simulink subsystem "digitalOutputs"  (R2023b)
settings: Solver=VariableStepAuto  StartTime=0.0  StopTime=10.0  RelTol=1e-3
settings Model: Creator=serga  LastModifiedBy=serga

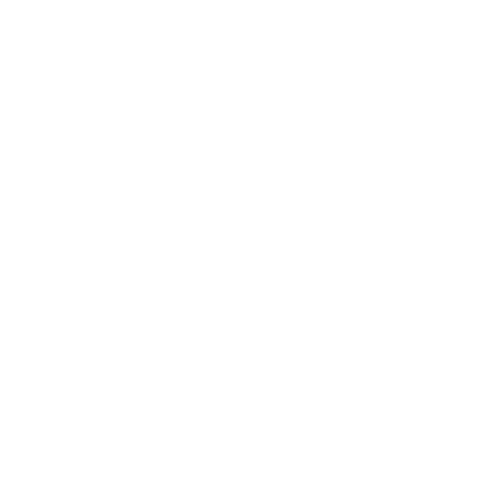
[thumbnail: Simulink's stored preview of the top-level diagram]
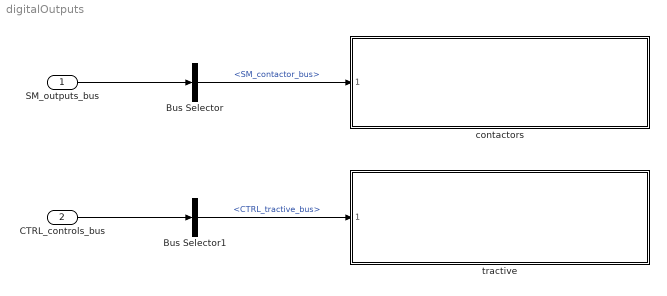
== system digitalOutputs ==
  SM_outputs_bus : Inport
  CTRL_controls_bus : Inport  Port=2
  Bus Selector : BusSelector  OutputSignals=SM_contactor_bus
  Bus Selector1 : BusSelector  OutputSignals=CTRL_tractive_bus
  contactors : Subsystem  ReferencedSubsystem=contactors
  tractive : Subsystem  ReferencedSubsystem=tractive
  wires:
  Bus Selector/1 -> contactors/1  "<SM_contactor_bus>"
  SM_outputs_bus/1 -> Bus Selector/1
  CTRL_controls_bus/1 -> Bus Selector1/1
  Bus Selector1/1 -> tractive/1  "<CTRL_tractive_bus>"
